simulink model "sampleModel48"  (R2021b)
settings: Solver=VariableStepAuto  StartTime=0.0  StopTime=10.0  RelTol=1e-3
undefined symbols (not defined in the file or in its folder): DiscIntNeverNeededParam, Newton, Raphson
libraries: simulink x5, slpidlib x1
settings Model: Creator=user  LastModifiedBy=user

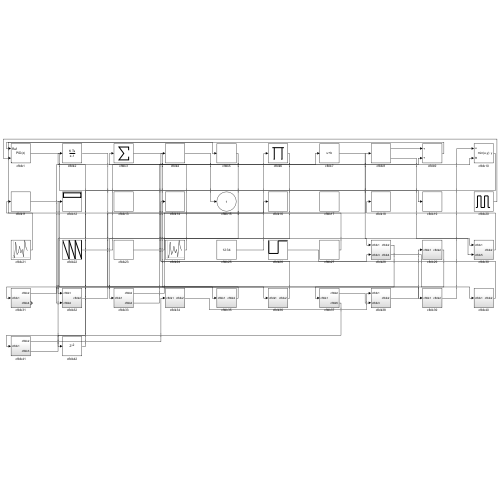
[thumbnail: Simulink's stored preview of the top-level diagram]
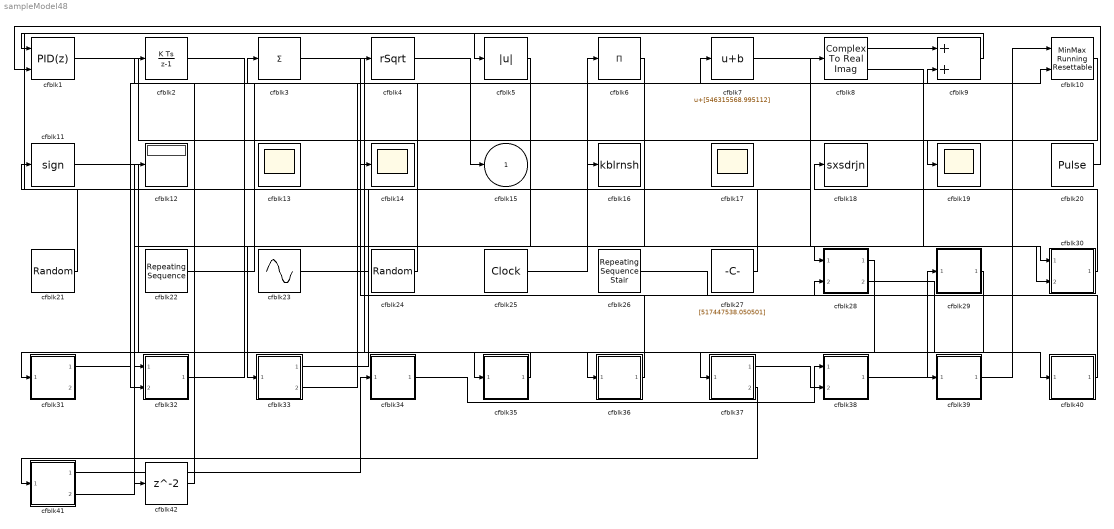
== system sampleModel48 ==
  cfblk1 : slpidlib/PID Controller (2DOF)  Controller=PID  Form=Parallel  TimeDomain=Discrete-time  UseExternalTs=off  SampleTime=1  IntegratorMethod=Forward Euler  FilterMethod=Forward Euler  ControllerParametersSource=internal  P=1  I=1  D=0  UseFilter=on  N=100  b=1  c=1  TunerSelectOption=Transfer Function Based (PID Tuner App)  InitialConditionSource=internal  InitialConditionForIntegrator=0  InitialConditionForFilter=0  DifferentiatorICPrevScaledInput=0  ExternalReset=none  TrackingMode=off  Kt=1  LimitOutput=off  SatLimitsSource=internal  UpperSaturationLimit=inf  LowerSaturationLimit=-inf  LinearizeAsGain=off  AntiWindupMode=none  Kb=1  POutMin=[]  POutMax=[]  IOutMin=[]  IOutMax=[]  DOutMin=[]  DOutMax=[]  NOutMin=[]  NOutMax=[]  bOutMin=[]  bOutMax=[]  cOutMin=[]  cOutMax=[]  SumOutMin=[]  SumOutMax=[]  SaturationOutMin=[]  SaturationOutMax=[]  PParamMin=[]  PParamMax=[]  IParamMin=[]  IParamMax=[]  DParamMin=[]  DParamMax=[]  NParamMin=[]  NParamMax=[]  bParamMin=[]  bParamMax=[]  cParamMin=[]  cParamMax=[]  KbParamMin=[]  KbParamMax=[]  KtParamMin=[]  KtParamMax=[]  KbOutMin=[]  KbOutMax=[]  KtOutMin=[]  KtOutMax=[]  IntegratorOutMin=[]  IntegratorOutMax=[]  FilterOutMin=[]  FilterOutMax=[]  SumI1OutMin=[]  SumI1OutMax=[]  SumI2OutMin=[]  SumI2OutMax=[]  SumI3OutMin=[]  SumI3OutMax=[]  SumI4OutMin=[]  SumI4OutMax=[]  SumDOutMin=[]  SumDOutMax=[]  Sum1OutMin=[]  Sum1OutMax=[]  Sum2OutMin=[]  Sum2OutMax=[]  Sum3OutMin=[]  Sum3OutMax=[]  DifferentiatorOutMin=[]  DifferentiatorOutMax=[]  FilterDiffOutCoefMin=[]  FilterDiffOutCoefMax=[]  ReciprocalOutMin=[]  ReciprocalOutMax=[]  SumDenOutMin=[]  SumDenOutMax=[]  SumNumOutMin=[]  SumNumOutMax=[]  DivideOutMin=[]  DivideOutMax=[]  UdiffTsProdOutMin=[]  UdiffTsProdOutMax=[]  NTsProdOutMin=[]  NTsProdOutMax=[]  UintegralTsProdOutMin=[]  UintegralTsProdOutMax=[]  UngainTsProdOutMin=[]  UngainTsProdOutMax=[]  IntegratorContinuousStateAttributes=''  IntegratorStateMustResolveToSignalObject=off  IntegratorRTWStateStorageClass=Auto  FilterContinuousStateAttributes=''  FilterStateMustResolveToSignalObject=off  FilterRTWStateStorageClass=Auto  ParallelPVariant=InternalParameters  IdealPVariant=Disabled  IVariant=InternalParameters  DVariant=InternalParameters  bVariant=InternalParameters  cVariant=InternalParameters  IntegratorVariant=Discrete  SatVariant=Disabled  AWVariant=Passthrough  PCopyVariant=Disabled  TRVariant=Disabled  FdbkBlocksVariant=Forward  IdealPFdbkVariant=Disabled  SatFdbkVariant=Disabled  DerivativeFilterVariant=ForwardEulerFilter  NVariant=InternalParameters  NCopyVariant=Disabled  FilterICVariant=InternalICsFilter  IntegratorICVariant=InternalICs  ExternalResetVariant=Disabled  TRSumVariant=Passthrough  SumFdbkVariant=Disabled  SumVariant=Sum_PID  TsampFilterVariant=InternalTs  TsampNgainVariant=Passthrough  TsampIntegralVariant=Passthrough  ExternalSaturationOutDataTypeStr=Inherit: Same as second input
      settings: SourceProductBaseCode=SL
  cfblk10 : simulink/Math Operations/MinMax Running Resettable  Function=min  vinit=0.0
  cfblk11 : Signum
  cfblk12 : Display
  cfblk{13..14,17,19} (4 alike) : Scope
      cfblk13 settings: Floating=on
      cfblk17 settings: Floating=on
  cfblk16 : ToWorkspace  VariableName=kblrnsh  SaveFormat=Timeseries  SampleTime=-1
  cfblk18 : ToWorkspace  VariableName=sxsdrjn  SaveFormat=Timeseries  SampleTime=-1
  cfblk2 : DiscreteIntegrator  ICPrevOutput=DiscIntNeverNeededParam  ICPrevScaledInput=DiscIntNeverNeededParam
  cfblk20 : DiscretePulseGenerator  PulseType=Time based  Amplitude=[-201982618.964050]  Period=[96043515.405813]  PulseWidth=5  PhaseDelay=[2.000000]
  cfblk21 : UniformRandomNumber  Minimum=[-4387808701.872269]  Maximum=[4672256919.373150]  Seed=[15893692.000000]  SampleTime=0.1
  cfblk22 : simulink/Sources/Repeating Sequence  rep_seq_t=[0 2]  rep_seq_y=[50395516.919247, -360520329.518330]
  cfblk23 : Sin  Amplitude=[562684814.290949]  Bias=[-874132188.809125]  SampleTime=0
  cfblk24 : UniformRandomNumber  Minimum=[-3776566144.895043]  Maximum=[6370537930.898802]  Seed=[8110523.000000]  SampleTime=0.1
  cfblk25 : DigitalClock
  cfblk26 : simulink/Sources/Repeating Sequence Stair  OutValues=[692628790.459985, 723871985.487427]  tsamp=-1  OutMin=[]  OutMax=[]  OutDataTypeStr=double  OutputDataTypeScalingMode=double  OutDataType=fixdt(0,8)  ConRadixGroup=Best Precision: Vector-wise  OutScaling=2^-12
  cfblk27 : Constant  Value=[517447538.050501]  SampleTime=1
  cfblk28 : Subsystem
  cfblk29 : Subsystem
  cfblk3 : Sum  Inputs=+
  cfblk30 : Subsystem
  cfblk31 : Subsystem
  cfblk32 : Subsystem
  cfblk33 : Subsystem
  cfblk34 : Subsystem
  cfblk35 : Subsystem
  cfblk36 : Subsystem
  cfblk37 : Subsystem
  cfblk38 : Subsystem
  cfblk39 : Subsystem
  cfblk4 : Sqrt  Operator=rSqrt  AlgorithmType=Newton-Raphson  SaturateOnIntegerOverflow=on
  cfblk40 : Subsystem
  cfblk41 : Subsystem
  cfblk42 : Delay  SampleTime=1
  cfblk5 : Abs
  cfblk6 : Product  Inputs=*
  cfblk7 : Bias  Bias=[546315568.995112]
  cfblk8 : ComplexToRealImag
  cfblk9 : Sum
  cfblk15 : Outport
  wires:
  cfblk1/1 -> cfblk19/1
  cfblk21/1 -> cfblk5/1
  cfblk11/1 -> cfblk35/1(cfblk1)
  cfblk23/1 -> cfblk28/1(cfblk1)
  cfblk41/1(cfblk2) -> cfblk34/1(cfblk1)
  cfblk4/1 -> cfblk15/1
  cfblk24/1 -> cfblk3/1
  cfblk39/1(cfblk2) -> cfblk10/1
  cfblk30/1(cfblk2) -> cfblk18/1
  cfblk28/1(cfblk2) -> cfblk37/1(cfblk1)
  cfblk28/2(cfblk4) -> cfblk40/1(cfblk1)
  cfblk41/2(cfblk3) -> cfblk12/1
  cfblk38/1(cfblk2) -> cfblk29/1(cfblk1)
  cfblk5/1 -> cfblk33/1(cfblk1)
  cfblk8/1 -> cfblk9/1
  cfblk27/1 -> cfblk11/1
  cfblk34/1(cfblk2) -> cfblk38/1(cfblk1)
  cfblk26/1 -> cfblk28/2(cfblk3)
  cfblk33/1(cfblk2) -> cfblk8/1
  cfblk35/1(cfblk2) -> cfblk31/1(cfblk1)
  cfblk2/1 -> cfblk39/1(cfblk1)
  cfblk7/1 -> cfblk30/1(cfblk1)
  cfblk37/1(cfblk2) -> cfblk38/2(cfblk3)
  cfblk3/1 -> cfblk36/1(cfblk1)
  cfblk22/1 -> cfblk10/2
  cfblk9/1 -> cfblk1/1
  cfblk20/1 -> cfblk1/2
  cfblk37/2(cfblk5) -> cfblk41/1(cfblk1)
  cfblk40/1(cfblk2) -> cfblk4/1
  cfblk6/1 -> cfblk32/1(cfblk1)
  cfblk33/2(cfblk4) -> cfblk9/2
  cfblk25/1 -> cfblk6/1
  cfblk36/1(cfblk2) -> cfblk14/1
  cfblk8/2 -> cfblk30/2(cfblk5)
  cfblk31/1(cfblk2) -> cfblk7/1
  cfblk32/1(cfblk2) -> cfblk16/1
  cfblk29/1(cfblk2) -> cfblk32/2(cfblk4)
  cfblk10/1 -> cfblk42/1
  cfblk42/1 -> cfblk2/1

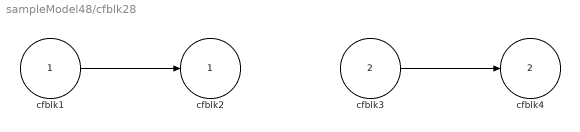
== system sampleModel48/cfblk28 ==
  cfblk1 : Inport
  cfblk3 : Inport  Port=2
  cfblk2 : Outport
  cfblk4 : Outport  Port=2
  wires:
  cfblk1/1 -> cfblk2/1
  cfblk3/1 -> cfblk4/1

== system sampleModel48/cfblk29 ==
  cfblk1 : Inport
  cfblk3 : DiscreteZeroPole  Poles=[0 0.5]  Gain=1
  cfblk2 : Outport
  wires:
  cfblk3/1 -> cfblk2/1
  cfblk1/1 -> cfblk3/1

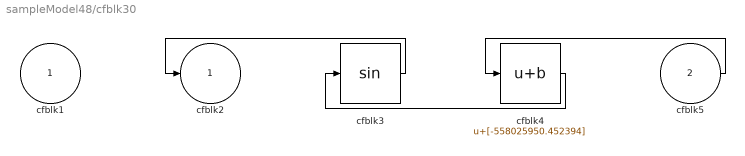
== system sampleModel48/cfblk30 ==
  cfblk1 : Inport
  cfblk5 : Inport  Port=2
  cfblk3 : Trigonometry
  cfblk4 : Bias  Bias=[-558025950.452394]
  cfblk2 : Outport
  wires:
  cfblk3/1 -> cfblk2/1
  cfblk5/1 -> cfblk4/1
  cfblk4/1 -> cfblk3/1

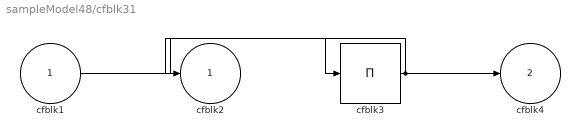
== system sampleModel48/cfblk31 ==
  cfblk1 : Inport
  cfblk3 : Product  Inputs=*
  cfblk2 : Outport
  cfblk4 : Outport  Port=2
  wires:
  cfblk1/1 -> cfblk3/1
  cfblk3/1 -> cfblk4/1, cfblk2/1

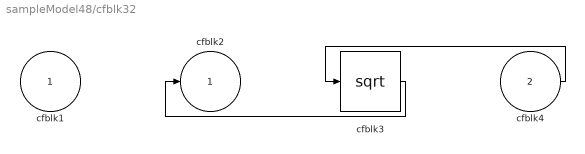
== system sampleModel48/cfblk32 ==
  cfblk1 : Inport
  cfblk4 : Inport  Port=2
  cfblk3 : Sqrt  SaturateOnIntegerOverflow=on
  cfblk2 : Outport
  wires:
  cfblk4/1 -> cfblk3/1
  cfblk3/1 -> cfblk2/1

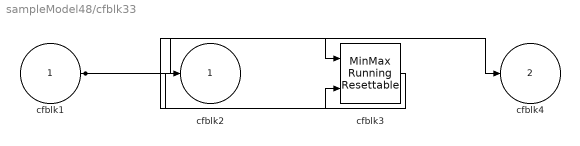
== system sampleModel48/cfblk33 ==
  cfblk1 : Inport
  cfblk3 : simulink/Math Operations/MinMax Running Resettable  Function=min  vinit=0.0
  cfblk2 : Outport
  cfblk4 : Outport  Port=2
  wires:
  cfblk1/1 -> cfblk4/1, cfblk3/1, cfblk3/2
  cfblk3/1 -> cfblk2/1

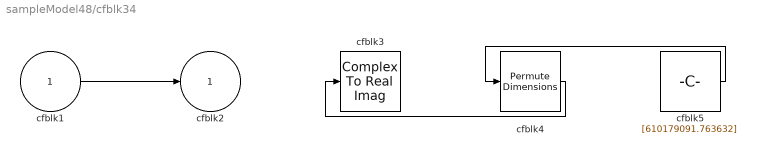
== system sampleModel48/cfblk34 ==
  cfblk1 : Inport
  cfblk3 : ComplexToRealImag
  cfblk4 : PermuteDimensions
  cfblk5 : Constant  Value=[610179091.763632]  SampleTime=1
  cfblk2 : Outport
  wires:
  cfblk5/1 -> cfblk4/1
  cfblk1/1 -> cfblk2/1
  cfblk4/1 -> cfblk3/1

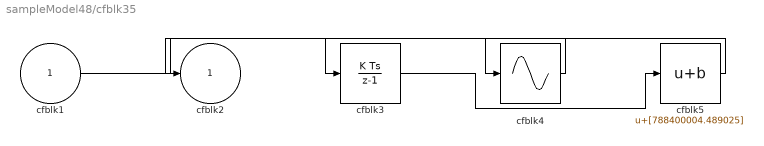
== system sampleModel48/cfblk35 ==
  cfblk1 : Inport
  cfblk3 : DiscreteIntegrator  ICPrevOutput=DiscIntNeverNeededParam  ICPrevScaledInput=DiscIntNeverNeededParam
  cfblk4 : Sin  TimeSource=Use external signal  SampleTime=0
  cfblk5 : Bias  Bias=[788400004.489025]
  cfblk2 : Outport
  wires:
  cfblk1/1 -> cfblk3/1
  cfblk5/1 -> cfblk4/1
  cfblk3/1 -> cfblk5/1
  cfblk4/1 -> cfblk2/1

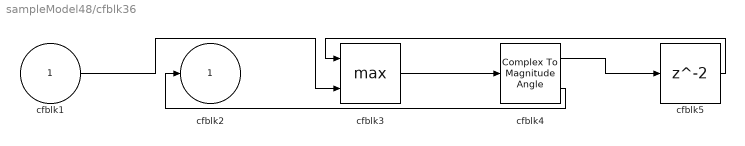
== system sampleModel48/cfblk36 ==
  cfblk1 : Inport
  cfblk3 : MinMax  Function=max  Inputs=2
  cfblk4 : ComplexToMagnitudeAngle
  cfblk5 : Delay  SampleTime=1
  cfblk2 : Outport
  wires:
  cfblk3/1 -> cfblk4/1
  cfblk4/2 -> cfblk2/1
  cfblk1/1 -> cfblk3/2
  cfblk4/1 -> cfblk5/1
  cfblk5/1 -> cfblk3/1

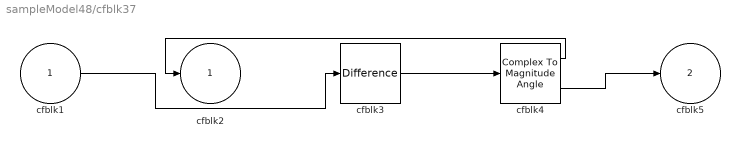
== system sampleModel48/cfblk37 ==
  cfblk1 : Inport
  cfblk3 : simulink/Discrete/Difference  ICPrevInput=0.0  OutMin=[]  OutMax=[]  OutDataTypeStr=Inherit: Inherit via back propagation  OutDataType=fixdt(1, 16)  OutScaling=2^-10  DoSatur=off
  cfblk4 : ComplexToMagnitudeAngle
  cfblk2 : Outport
  cfblk5 : Outport  Port=2
  wires:
  cfblk4/1 -> cfblk2/1
  cfblk4/2 -> cfblk5/1
  cfblk3/1 -> cfblk4/1
  cfblk1/1 -> cfblk3/1

== system sampleModel48/cfblk38 ==
  cfblk1 : Inport
  cfblk3 : Inport  Port=2
  cfblk2 : Outport
  wires:
  cfblk3/1 -> cfblk2/1

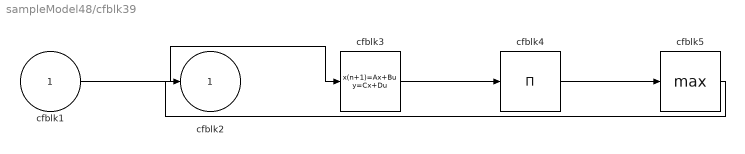
== system sampleModel48/cfblk39 ==
  cfblk1 : Inport
  cfblk3 : DiscreteStateSpace
  cfblk4 : Product  Inputs=*
  cfblk5 : MinMax  Function=max
  cfblk2 : Outport
  wires:
  cfblk1/1 -> cfblk3/1
  cfblk3/1 -> cfblk4/1
  cfblk5/1 -> cfblk2/1
  cfblk4/1 -> cfblk5/1

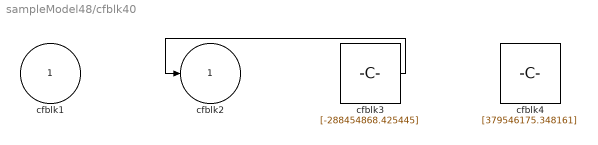
== system sampleModel48/cfblk40 ==
  cfblk1 : Inport
  cfblk3 : Constant  Value=[-288454868.425445]  SampleTime=1
  cfblk4 : Constant  Value=[379546175.348161]  SampleTime=1
  cfblk2 : Outport
  wires:
  cfblk3/1 -> cfblk2/1

== system sampleModel48/cfblk41 ==
  cfblk1 : Inport
  cfblk2 : Outport
  cfblk3 : Outport  Port=2
  wires:
  cfblk1/1 -> cfblk2/1, cfblk3/1
